simulink model "model"  (R2024a)
settings: Solver=VariableStepAuto  StartTime=0.0  StopTime=10.0  FixedStep=0.0001  RelTol=1e-3
values from neighbouring files (symbols this model uses):
  d1 = exp(-T/T1)    [calc.m]    (also in first_calc.m)
  d2 = exp(-T/T2)    [calc.m]    (also in first_calc.m)
  q0 = 18    [calc.m]    (also in first_calc.m = 2)
  T = T1/2    (= 0.225)    [calc.m]    (also in first_calc.m; second_calc.m = 0.2)
  T1 = 0.45    [calc.m]    (also in first_calc.m)
  T2_1 = 1.2*1.35    (= 1.62)    [calc.m]
libraries: simulink x1
settings Model: Creator=ventus  LastModifiedBy=ventus

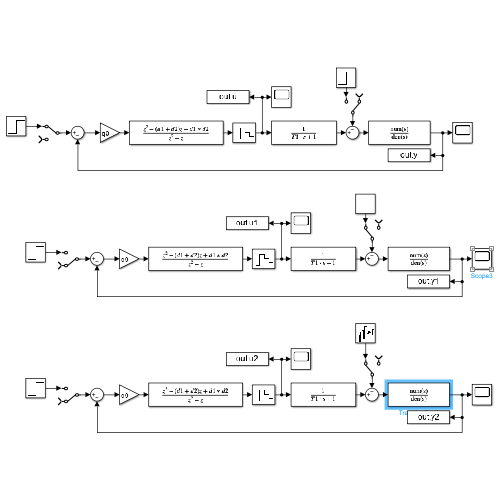
[thumbnail: Simulink's stored preview of the top-level diagram]
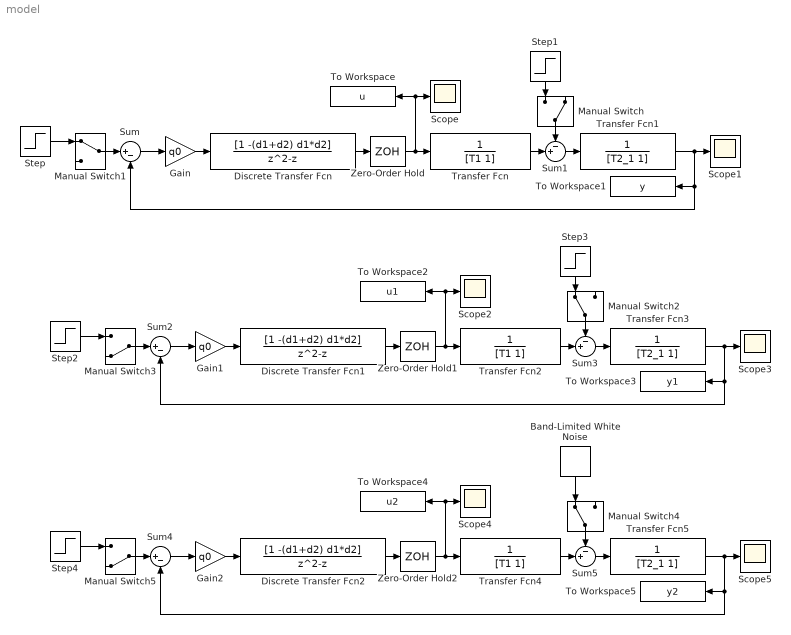
== system model ==
  Band-Limited White Noise : simulink/Sources/Band-Limited White Noise  Cov=[0.1]  Ts=T  seed=[23341]
  Discrete Transfer Fcn : DiscreteTransferFcn  Numerator=[1 -(d1+d2) d1*d2]  Denominator=[1 -1 0]
  Discrete Transfer Fcn1 : DiscreteTransferFcn  Numerator=[1 -(d1+d2) d1*d2]  Denominator=[1 -1 0]
  Discrete Transfer Fcn2 : DiscreteTransferFcn  Numerator=[1 -(d1+d2) d1*d2]  Denominator=[1 -1 0]
  Gain : Gain  Gain=q0
  Gain1 : Gain  Gain=q0
  Gain2 : Gain  Gain=q0
  Manual Switch : ManualSwitch  CurrentSetting=0
  Manual Switch1 : ManualSwitch
  Manual Switch2 : ManualSwitch
  Manual Switch3 : ManualSwitch  CurrentSetting=0
  Manual Switch4 : ManualSwitch
  Manual Switch5 : ManualSwitch  CurrentSetting=0
  Scope{,1..5} (6 alike) : Scope
  Step{,1..4} (5 alike) : Step  SampleTime=0
  Sum : Sum  Inputs=|+-
  Sum1 : Sum  Inputs=-+|
  Sum2 : Sum  Inputs=|+-
  Sum3 : Sum  Inputs=-+|
  Sum4 : Sum  Inputs=|+-
  Sum5 : Sum  Inputs=-+|
  To Workspace : ToWorkspace  VariableName=u  SaveFormat=Timeseries  SampleTime=-1
  To Workspace1 : ToWorkspace  VariableName=y  SaveFormat=Timeseries  SampleTime=-1
  To Workspace2 : ToWorkspace  VariableName=u1  SaveFormat=Timeseries  SampleTime=-1
  To Workspace3 : ToWorkspace  VariableName=y1  SaveFormat=Timeseries  SampleTime=-1
  To Workspace4 : ToWorkspace  VariableName=u2  SaveFormat=Timeseries  SampleTime=-1
  To Workspace5 : ToWorkspace  VariableName=y2  SaveFormat=Timeseries  SampleTime=-1
  Transfer Fcn : TransferFcn  Denominator=[T1 1]
  Transfer Fcn1 : TransferFcn  Denominator=[T2_1 1]
  Transfer Fcn2 : TransferFcn  Denominator=[T1 1]
  Transfer Fcn3 : TransferFcn  Denominator=[T2_1 1]
  Transfer Fcn4 : TransferFcn  Denominator=[T1 1]
  Transfer Fcn5 : TransferFcn  Denominator=[T2_1 1]
  Zero-Order Hold : ZeroOrderHold  SampleTime=T
  Zero-Order Hold1 : ZeroOrderHold  SampleTime=T
  Zero-Order Hold2 : ZeroOrderHold  SampleTime=T
  wires:
  Step/1 -> Manual Switch1/1
  Manual Switch1/1 -> Sum/1
  Sum/1 -> Gain/1
  Zero-Order Hold/1 -> To Workspace/1, Scope/1, Transfer Fcn/1
  Transfer Fcn/1 -> Sum1/2
  Manual Switch/1 -> Sum1/1
  Step1/1 -> Manual Switch/1
  Sum1/1 -> Transfer Fcn1/1
  Transfer Fcn1/1 -> Scope1/1, To Workspace1/1, Sum/2
  Discrete Transfer Fcn/1 -> Zero-Order Hold/1
  Gain/1 -> Discrete Transfer Fcn/1
  Gain1/1 -> Discrete Transfer Fcn1/1
  Transfer Fcn2/1 -> Sum3/2
  Manual Switch3/1 -> Sum2/1
  Sum2/1 -> Gain1/1
  Zero-Order Hold1/1 -> To Workspace2/1, Scope2/1, Transfer Fcn2/1
  Discrete Transfer Fcn1/1 -> Zero-Order Hold1/1
  Step3/1 -> Manual Switch2/1
  Transfer Fcn3/1 -> Scope3/1, To Workspace3/1, Sum2/2
  Manual Switch2/1 -> Sum3/1
  Sum3/1 -> Transfer Fcn3/1
  Step2/1 -> Manual Switch3/1
  Gain2/1 -> Discrete Transfer Fcn2/1
  Transfer Fcn4/1 -> Sum5/2
  Manual Switch5/1 -> Sum4/1
  Sum4/1 -> Gain2/1
  Zero-Order Hold2/1 -> To Workspace4/1, Scope4/1, Transfer Fcn4/1
  Discrete Transfer Fcn2/1 -> Zero-Order Hold2/1
  Transfer Fcn5/1 -> Scope5/1, To Workspace5/1, Sum4/2
  Manual Switch4/1 -> Sum5/1
  Sum5/1 -> Transfer Fcn5/1
  Step4/1 -> Manual Switch5/1
  Band-Limited White Noise/1 -> Manual Switch4/1
